simulink model "SBFSRM_CustomModelOK_WindTurbine_1Hp"  (Simulink 8.1)
settings: Solver=ode45  StartTime=0.0  StopTime=0.5  FixedStep=Ts  MaxStep=1e-6  MinStep=1e-7  RelTol=1e-5
values from neighbouring files (symbols this model uses):
  Bm = 0.02    [WorkSpaceBackup1.mat]
  J = 0.048    [WorkSpaceBackup1.mat]
  R = 0.05    [WorkSpaceBackup1.mat]
  Ts = 1e-06    [WorkSpaceBackup1.mat]
undefined symbols (not defined in the file or in its folder): DiscIntNeverNeededParam, find_system, InductanceTest, TorqueTest
libraries: powerlib x49, powerlib_extras x2, simulink x2, dspsigops x1
settings Model: Creator=Rahul  LastModifiedBy=USER
settings DataIOCC: SignalLoggingName=signout
settings OptimizationCC: InitFltsAndDblsToZero=on
settings DebuggingCC: CheckExecutionContextPreStartOutputMsg=on  CheckExecutionContextRuntimeOutputMsg=on  SolverPrmCheckMsg=none  MultiTaskDSMMsg=warning  MultiTaskCondExecSysMsg=none
settings HardwareCC: TargetHWDeviceType=32-bit Generic

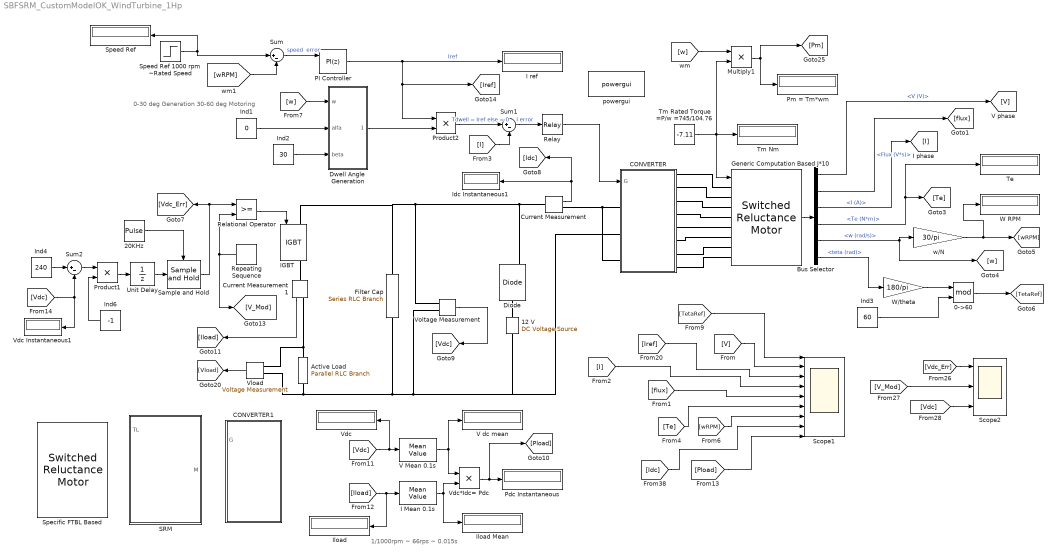
== system SBFSRM_CustomModelOK_WindTurbine_1Hp ==
  note: 1/1000rpm ~ 66rps ~ 0.015s
  note: 0-30 deg Generation
      | 30-60 deg Motoring
  0->60 : Math  Operator=mod  SampleTime=Ts  SaturateOnIntegerOverflow=on
  12 V : powerlib/Electrical Sources/DC Voltage Source  Amplitude=200  Measurements=None
  20KHz : DiscretePulseGenerator  PulseType=Time based  Period=0.5e-4  PulseWidth=10
  Active Load : powerlib/Elements/Parallel RLC Branch  LConnTagsString=a  RConnTagsString=__new0  BranchType=R  Resistance=1  Inductance=1e-3  SetiL0=off  InitialCurrent=0  Capacitance=1e-6  Setx0=off  InitialVoltage=0  Measurements=None
  Bus Selector : BusSelector  OutputSignals=V (V),Flux (V*s),I (A),Te (N*m),w (rad/s),teta (rad)
  CONVERTER : Subsystem  LoadFcn=find_system(gcs,'FollowLinks', 'on', 'LookUnderMasks', 'all');
  CONVERTER1 : Subsystem  LoadFcn=find_system(gcs,'FollowLinks', 'on', 'LookUnderMasks', 'all');
  Current Measurement : powerlib/Measurements/Current Measurement  PhasorSimulation=off  OutputType=Complex  PSBequivalent=0
  Current Measurement1 : powerlib/Measurements/Current Measurement  PhasorSimulation=off  OutputType=Complex  PSBequivalent=0
  Diode : powerlib/Power Electronics/Diode  Ron=0.001  Lon=0  Vf=0.8  IC=0  UseSnubber=off  Rs=10e6  Cs=inf  Measurements=on
  Dwell Angle  Generation : Subsystem
  Filter Cap : powerlib/Elements/Series RLC Branch  LConnTagsString=__new0  RConnTagsString=__new0  BranchType=RC  Resistance=0.001  Inductance=1e-3  SetiL0=off  InitialCurrent=0  Capacitance=3000e-6  Setx0=off  InitialVoltage=0  Measurements=None
  "Generic Computation Based J*10 " : powerlib/Machines/Switched Reluctance Motor  MachineType=8/6  MachineModel=Generic model  StatorResistance=0.013  PlotCurves=off  Inertia=0.0004  Friction=0  InitialSpeed=[97 0]  Lq=0.005  Ld=0.053  Lsat=0.002  MaximumCurrent=20  MaximumFluxLinkage=0.3  MagnetisationCharacteristic='srm64_60kw.mat'  RotorAngleVector=[0 10 20 30 40 45]  StatorCurrentVector=0:25:450  TsPowergui=0  TsBlock=-1
  I Mean 0.1s : powerlib_extras/Measurements/Mean Value  Period=0.015
  I ref : Display
  IGBT : powerlib/Power Electronics/IGBT  Ron=0.001  Lon=0  Vf=1  Tf=1e-6  Tt=2e-6  IC=0  Rs=1e5  Cs=inf  Measurements=on
  Idc Instantaneous1 : Display
  "Iload " : Display
  Iload Mean : Display
  Ind1 : Constant  Value=0
  Ind2 : Constant  Value=30
  Ind3 : Constant  Value=60
  Ind4 : Constant  Value=240
  Ind6 : Constant  Value=-1
  Multiply1 : Product  Inputs=**
  PI Controller : simulink/Continuous/PID Controller  Controller=PI  TimeDomain=Discrete-time  SampleTime=Ts  IntegratorMethod=Trapezoidal  FilterMethod=Forward Euler  Form=Parallel  P=-2  I=-0.1  D=0  N=100  InitialConditionSource=external  InitialConditionForIntegrator=0  InitialConditionForFilter=0  ExternalReset=none  LimitOutput=on  UpperSaturationLimit=20  LowerSaturationLimit=0  LinearizeAsGain=off  AntiWindupMode=clamping  Kb=1  TrackingMode=off  Kt=1  PParamMin=[]  PParamMax=[]  IParamMin=[]  IParamMax=[]  DParamMin=[]  DParamMax=[]  NParamMin=[]  NParamMax=[]  KbParamMin=[]  KbParamMax=[]  KtParamMin=[]  KtParamMax=[]  POutMin=[]  POutMax=[]  IOutMin=[]  IOutMax=[]  DOutMin=[]  DOutMax=[]  NOutMin=[]  NOutMax=[]  KbOutMin=[]  KbOutMax=[]  KtOutMin=[]  KtOutMax=[]  IntegratorOutMin=[]  IntegratorOutMax=[]  FilterOutMin=[]  FilterOutMax=[]  SumOutMin=[]  SumOutMax=[]  SumI1OutMin=[]  SumI1OutMax=[]  SumI2OutMin=[]  SumI2OutMax=[]  SumI3OutMin=[]  SumI3OutMax=[]  SumDOutMin=[]  SumDOutMax=[]  SaturationOutMin=[]  SaturationOutMax=[]  IntegratorContinuousStateAttributes=''  IntegratorStateMustResolveToSignalObject=off  IntegratorRTWStateStorageClass=Auto  FilterContinuousStateAttributes=''  FilterStateMustResolveToSignalObject=off  FilterRTWStateStorageClass=Auto
  Pdc Instantaneous : Display
  Pm = Tm*wm : Display
  Product1 : Product
  Product2 : Product  RndMeth=Zero
  Relational Operator : RelationalOperator  OutDataTypeStr=boolean
  Relay : Relay  OnSwitchValue=0.1  OffSwitchValue=-0.1
  Repeating Sequence : simulink/Sources/Repeating Sequence  rep_seq_t=[0 0.25e-4 0.5e-4]  rep_seq_y=[0 1 0]
  SRM : Subsystem
  Sample and Hold : dspsigops/Sample and Hold  trig=Rising edge  initCond=0  latchinput=off
  Scope1 : Scope  NumInputPorts=9
      settings: TimeRange=0.1400000000000001  YMin=0~-300~0~-5~-0.1~-10~0~-250~0  YMax=100~300~12~20~0.4~10~1200~250~800  SaveName=ScopeData2  MaxDataPoints=100000
  Scope2 : Scope  NumInputPorts=3
      settings: TimeRange=0.1400000000000001  YMin=-5~-2~0  YMax=5~2~300  MaxDataPoints=100000
  Specific FTBL Based : powerlib/Machines/Switched Reluctance Motor  MachineType=6/4  MachineModel=Specific model  StatorResistance=R  PlotCurves=off  Inertia=J  Friction=Bm  InitialSpeed=[355 0]  Lq=0.67e-3  Ld=23.6e-3  Lsat=0.15e-3  MaximumCurrent=450  MaximumFluxLinkage=0.486  MagnetisationCharacteristic='SRM64StandardTables.mat'  RotorAngleVector=[0,1,2,3,4,5,6,7,8,9,10,11,12,13,14,15,16,17,18,19,20,21,22,23,24,25,26,27,28,29,30,31,32,33,34,35,36,37,38,39,40,41,42,43,44,45,46,47,48,49,50,51,52,53,54,55,56,57,58,59,60,61,62,63,64,65,66,67,68,69,70,71,72,73,74,75,76,77,78,79,80,81,82,83,84,85,86,87,88,89,90]  StatorCurrentVector=[0,0.1,0.3,0.5,0.7,0.9,1,2,3,4,5,6,7,8,9,10,11,12,13,14,15,16,17,18,19,20,21,22,23,24,25,26,27,28,29,30,31,32,33,34,35,36,37,38,39,40,41,42,43,44,45,46,47,48,49,50,51,52,53,54,55,56,57,58,59,60,61,62,63,64,65,66,67,68,69,70,71,72,73,74,75,76,77,78,79,80,81,82,83,84,85,86,87,88,89,90,91,92,93,94,95,96,97,98,99,100,101,102,103,104,105,106,107,108,109,110,111,112,113,114,115,116,117,118,119,120,121,122,123,124,125,126,127,128,129,130,131,132,133,134,135,136,137,138,139,140,141,142,143,144,145,146,147,148,149,150,151,152,153,154,155,156,157,158,159,160,161,162,163,164,165,166,167,168]  TsPowergui=0  TsBlock=-1
  Speed Ref : Display
  Speed Ref 1000 rpm ~Rated Speed : Step  Time=0.1  Before=1000  After=1000  SampleTime=0
  Sum : Sum  Inputs=|+-
  Sum1 : Sum  Inputs=|+-
  Sum2 : Sum  Inputs=|+-
  Te : Display
  Tm Nm : Display
  Tm Rated Torque =P/w =745/104.76 : Constant  Value=-7.11
  Unit Delay : UnitDelay  SampleTime=-1
  V Mean 0.1s : powerlib_extras/Measurements/Mean Value  Period=0.015
  V dc mean : Display
  "Vdc " : Display
  Vdc Instantaneous1 : Display
  Vdc*Idc= Pdc : Product
  Vload : powerlib/Measurements/Voltage Measurement  PhasorSimulation=off  OutputType=Complex  PSBequivalent=0
  Voltage Measurement : powerlib/Measurements/Voltage Measurement  PhasorSimulation=off  OutputType=Complex  PSBequivalent=0
  W RPM : Display
  W/theta : Gain  Gain=180/pi
  powergui : powerlib/powergui  Priority=1  SimulationMode=Discrete  SolverType=Tustin  SampleTime=Ts  frequency=60  SPID=off  DisableSnubberDevices=off  DisableRonSwitches=off  DisableVfSwitches=off  SwTol=0  Interpol=off  DisplayEquations=off  frequencyindice=0  Pbase=100e6  ErrMax=1e-4  Iterations=50  UnitsV=kV  UnitsW=MW  FunctionMessages=off  echomessages=off  HookPort=off  EnableUseOfTLC=off  x0status=blocks  RestoreLinks=warning  ResistiveCurrentMeasurement=off  Frange=[0:2:500]  Ylog=off  Xlog=on  ShowGrid=off  save=off  variable=ZData  ZoomFFT=off  StartTime=0.0  cycles=1  DisplayStyle=1  fundamental=60  FreqAxis=off  MaxFrequency=1000  frequencyindicesteady=1  RmsSteady=1  display=off  Ts=0  methode=off
  w/N : Gain  Gain=30/pi
  wires:
  Sum1/1 -> Relay/1  "I error"
  Relay/1 -> CONVERTER/1(G)
  Product2/1 -> Sum1/1  "Tdwell = Iref else = 0"
  "Generic Computation Based J*10 "/1 -> Bus Selector/1
  Bus Selector/6 -> W/theta/1  "<teta (rad)>"
  w/N/1 -> [wRPM], W RPM/1
  Ind3/1 -> 0->60/2
  W/theta/1 -> 0->60/1
  Bus Selector/1 -> [V]  "<V (V)>"
  Bus Selector/2 -> [flux]  "<Flux (V*s)>"
  Bus Selector/3 -> [I]  "<I (A)>"
  [I] -> Sum1/2
  Bus Selector/4 -> [Te], Te/1  "<Te (N*m)>"
  Bus Selector/5 -> w/N/1, [w]  "<w (rad/s)>"
  0->60/1 -> [TetaRef]
  Voltage Measurement/1 -> [Vdc]
  Current Measurement/1 -> Idc Instantaneous1/1, [Idc]
  [Iload] -> I Mean 0.1s/1, "Iload "/1
  Ind4/1 -> Sum2/1
  [Vdc] -> Sum2/2, Vdc Instantaneous1/1
  Vdc*Idc= Pdc/1 -> [Pload], Pdc Instantaneous/1
  Current Measurement1/1 -> [Iload]
  [w] -> Multiply1/1
  Multiply1/1 -> [Pm], Pm = Tm*wm/1
  Tm Rated Torque =P/w =745/104.76/1 -> Tm Nm/1, "Generic Computation Based J*10 "/1, Multiply1/2
  Repeating Sequence/1 -> Relational Operator/2, [V_Mod]
  Relational Operator/1 -> IGBT/1
  Sum2/1 -> Product1/1
  Ind6/1 -> Product1/2
  Product1/1 -> Unit Delay/1
  Unit Delay/1 -> Sample and Hold/1
  Sample and Hold/1 -> Relational Operator/1, [Vdc_Err]
  20KHz/1 -> Sample and Hold/Trigger
  [Vdc] -> V Mean 0.1s/1, "Vdc "/1
  I Mean 0.1s/1 -> Iload Mean/1, Vdc*Idc= Pdc/2
  Vload/1 -> [Vload]
  V Mean 0.1s/1 -> V dc mean/1, Vdc*Idc= Pdc/1
  Ind1/1 -> Dwell Angle  Generation/2(alfa)
  Ind2/1 -> Dwell Angle  Generation/3(beta)
  [w] -> Dwell Angle  Generation/1(w)
  Dwell Angle  Generation/1(Signal) -> Product2/2
  [TetaRef] -> Scope1/1
  [V] -> Scope1/2
  [Iref] -> Scope1/3
  [I] -> Scope1/4
  [Pload] -> Scope1/9
  [Idc] -> Scope1/8
  [wRPM] -> Scope1/7
  [Te] -> Scope1/6
  [flux] -> Scope1/5
  [Vdc_Err] -> Scope2/1
  [V_Mod] -> Scope2/2
  [Vdc] -> Scope2/3
  Sum/1 -> PI Controller/1  "speed  error"
  Speed Ref 1000 rpm ~Rated Speed/1 -> Sum/1, Speed Ref/1
  [wRPM] -> Sum/2
  PI Controller/1 -> Product2/1, [Iref], I ref/1  "Iref"
  connections:
  "Generic Computation Based J*10 "/LConn1 -- CONVERTER/RConn1
  "Generic Computation Based J*10 "/LConn2 -- CONVERTER/RConn2
  "Generic Computation Based J*10 "/LConn3 -- CONVERTER/RConn3
  "Generic Computation Based J*10 "/LConn4 -- CONVERTER/RConn4
  "Generic Computation Based J*10 "/LConn5 -- CONVERTER/RConn5
  "Generic Computation Based J*10 "/LConn6 -- CONVERTER/RConn6
  Voltage Measurement/LConn2 -- Vload/LConn2 -- Active Load/RConn1 -- Filter Cap/RConn1 -- CONVERTER/LConn2 -- 12 V/LConn1
  Current Measurement/LConn1 -- Filter Cap/LConn1 -- IGBT/LConn1 -- Voltage Measurement/LConn1 -- Diode/RConn1
  Current Measurement/RConn1 -- CONVERTER/LConn3 -- CONVERTER/LConn1
  Diode/LConn1 -- 12 V/RConn1
  Active Load/LConn1 -- Vload/LConn1 -- Current Measurement1/RConn1
  IGBT/RConn1 -- Current Measurement1/LConn1
  CONVERTER/RConn7 -- "Generic Computation Based J*10 "/LConn7
  CONVERTER/RConn8 -- "Generic Computation Based J*10 "/LConn8

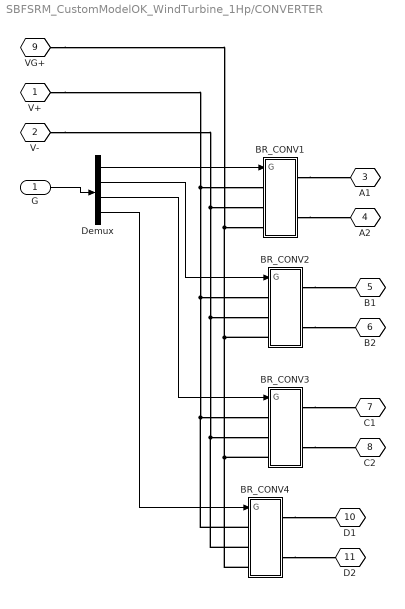
== system SBFSRM_CustomModelOK_WindTurbine_1Hp/CONVERTER ==
  G : Inport
  BR_CONV1 : Subsystem
  BR_CONV2 : Subsystem
  BR_CONV3 : Subsystem
  BR_CONV4 : Subsystem
  Demux : Demux
  V+ : PMIOPort  Tag=PMCPort  Port=1  Side=Left
  V- : PMIOPort  Tag=PMCPort  Port=2  Side=Left
  A1 : PMIOPort  Tag=PMCPort  Port=3  Side=Right
  A2 : PMIOPort  Tag=PMCPort  Port=4  Side=Right
  B1 : PMIOPort  Tag=PMCPort  Port=5  Side=Right
  B2 : PMIOPort  Tag=PMCPort  Port=6  Side=Right
  C1 : PMIOPort  Tag=PMCPort  Port=7  Side=Right
  C2 : PMIOPort  Tag=PMCPort  Port=8  Side=Right
  VG+ : PMIOPort  Tag=PMCPort  Port=9  Side=Left
  D1 : PMIOPort  Tag=PMCPort  Port=10  Side=Right
  D2 : PMIOPort  Tag=PMCPort  Port=11  Side=Right
  wires:
  Demux/3 -> BR_CONV3/1(G)
  Demux/1 -> BR_CONV1/1(G)
  G/1 -> Demux/1
  Demux/2 -> BR_CONV2/1(G)
  Demux/4 -> BR_CONV4/1(G)
  connections:
  BR_CONV3/RConn2 -- C2/RConn1
  BR_CONV3/RConn1 -- C1/RConn1
  BR_CONV2/RConn2 -- B2/RConn1
  BR_CONV2/RConn1 -- B1/RConn1
  BR_CONV1/RConn2 -- A2/RConn1
  BR_CONV1/RConn1 -- A1/RConn1
  BR_CONV1/LConn2 -- V-/RConn1 -- BR_CONV4/LConn2 -- BR_CONV3/LConn2 -- BR_CONV2/LConn2
  V+/RConn1 -- BR_CONV1/LConn1 -- BR_CONV4/LConn1 -- BR_CONV3/LConn1 -- BR_CONV2/LConn1
  VG+/RConn1 -- BR_CONV1/LConn3 -- BR_CONV4/LConn3 -- BR_CONV3/LConn3 -- BR_CONV2/LConn3
  BR_CONV4/RConn2 -- D2/RConn1
  BR_CONV4/RConn1 -- D1/RConn1

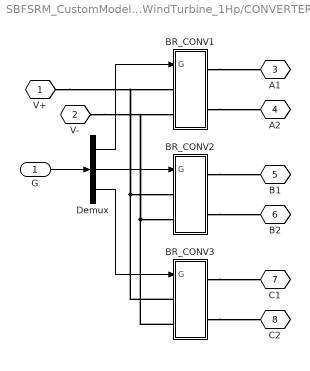
== system SBFSRM_CustomModelOK_WindTurbine_1Hp/CONVERTER1 ==
  G : Inport
  BR_CONV1 : Subsystem
  BR_CONV2 : Subsystem
  BR_CONV3 : Subsystem
  Demux : Demux  Outputs=3
  V+ : PMIOPort  Tag=PMCPort  Port=1  Side=Left
  V- : PMIOPort  Tag=PMCPort  Port=2  Side=Left
  A1 : PMIOPort  Tag=PMCPort  Port=3  Side=Right
  A2 : PMIOPort  Tag=PMCPort  Port=4  Side=Right
  B1 : PMIOPort  Tag=PMCPort  Port=5  Side=Right
  B2 : PMIOPort  Tag=PMCPort  Port=6  Side=Right
  C1 : PMIOPort  Tag=PMCPort  Port=7  Side=Right
  C2 : PMIOPort  Tag=PMCPort  Port=8  Side=Right
  wires:
  Demux/3 -> BR_CONV3/1(G)
  Demux/1 -> BR_CONV1/1(G)
  Demux/2 -> BR_CONV2/1(G)
  G/1 -> Demux/1
  connections:
  BR_CONV3/RConn2 -- C2/RConn1
  BR_CONV3/RConn1 -- C1/RConn1
  BR_CONV2/RConn2 -- B2/RConn1
  BR_CONV2/RConn1 -- B1/RConn1
  BR_CONV1/RConn2 -- A2/RConn1
  BR_CONV1/RConn1 -- A1/RConn1
  BR_CONV3/LConn2 -- BR_CONV1/LConn2 -- V-/RConn1 -- BR_CONV2/LConn2
  BR_CONV3/LConn1 -- BR_CONV1/LConn1 -- V+/RConn1 -- BR_CONV2/LConn1

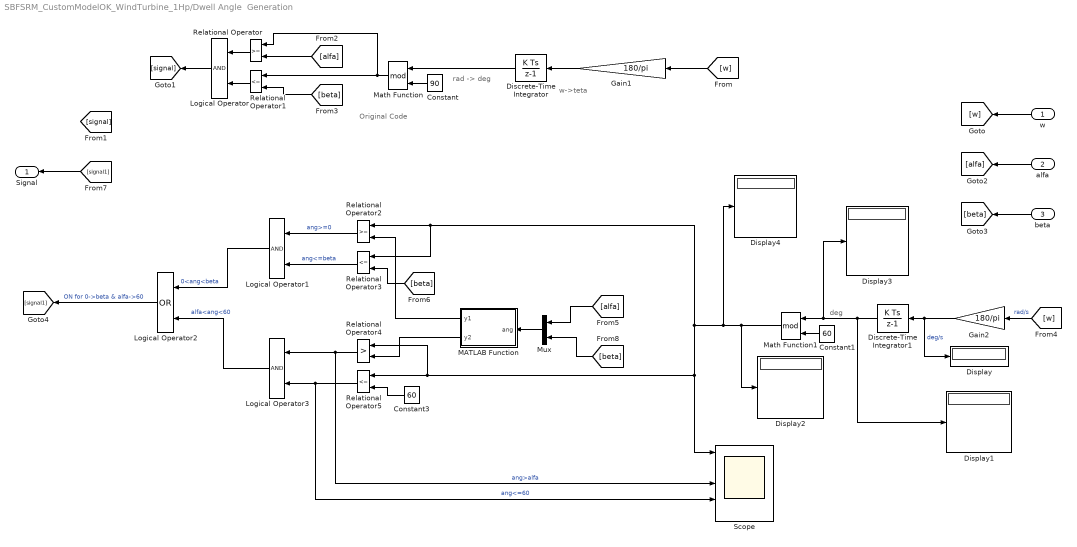
== system SBFSRM_CustomModelOK_WindTurbine_1Hp/Dwell Angle  Generation ==
  note: Original Code
  note: rad -> deg
  note: w->teta
  note: deg
  w : Inport
  alfa : Inport  Port=2
  beta : Inport  Port=3
  Constant : Constant  Value=90
  Constant1 : Constant  Value=60
  Constant3 : Constant  Value=60
  Discrete-Time Integrator : DiscreteIntegrator  InitialCondition=[0 -30 -60]  SampleTime=Ts  ICPrevOutput=DiscIntNeverNeededParam  ICPrevScaledInput=DiscIntNeverNeededParam
  Discrete-Time Integrator1 : DiscreteIntegrator  InitialCondition=[0 -15 -30 -45]  SampleTime=Ts  ICPrevOutput=DiscIntNeverNeededParam  ICPrevScaledInput=DiscIntNeverNeededParam
  Display{,1..4} (5 alike) : Display
  Gain1 : Gain  Gain=180/pi  SaturateOnIntegerOverflow=on  OutDataTypeStr=Inherit: Same as input  ParamDataTypeStr=Inherit: Same as input
  Gain2 : Gain  Gain=180/pi  SaturateOnIntegerOverflow=on  OutDataTypeStr=Inherit: Same as input  ParamDataTypeStr=Inherit: Same as input
  Logical Operator : Logic  AllPortsSameDT=off
  Logical Operator1 : Logic  AllPortsSameDT=off
  Logical Operator2 : Logic  Operator=OR  AllPortsSameDT=off
  Logical Operator3 : Logic  AllPortsSameDT=off
  MATLAB Function : MATLAB Function  TreatAsAtomicUnit=on
  Math Function : Math  Operator=mod  SaturateOnIntegerOverflow=on
  Math Function1 : Math  Operator=mod  SaturateOnIntegerOverflow=on
  Mux : Mux  Inputs=2
  Relational Operator : RelationalOperator
  Relational Operator1 : RelationalOperator  Operator=<=
  Relational Operator2 : RelationalOperator
  Relational Operator3 : RelationalOperator  Operator=<=
  Relational Operator4 : RelationalOperator  Operator=>
  Relational Operator5 : RelationalOperator  Operator=<=
  Scope : Scope  NumInputPorts=5
      settings: YMin=-5~-5~-5~-5~-5  YMax=5~5~5~5~5
  Signal : Outport
  wires:
  Math Function/1 -> Relational Operator/1, Relational Operator1/1
  Relational Operator1/1 -> Logical Operator/2
  beta/1 -> [beta]
  alfa/1 -> [alfa]
  Relational Operator/1 -> Logical Operator/1
  Constant/1 -> Math Function/2
  Logical Operator/1 -> [signal]
  Discrete-Time Integrator/1 -> Math Function/1
  Gain1/1 -> Discrete-Time Integrator/1
  w/1 -> [w]
  [w] -> Gain2/1  "rad/s"
  Math Function1/1 -> Display2/1, Relational Operator3/1, Relational Operator2/1, Scope/1, Relational Operator4/1, Relational Operator5/1, Display4/1
  Gain2/1 -> Display/1, Discrete-Time Integrator1/1  "deg/s"
  [beta] -> Relational Operator3/2
  Relational Operator2/1 -> Logical Operator1/1  "ang>=0"
  Constant1/1 -> Math Function1/2
  Discrete-Time Integrator1/1 -> Display1/1, Math Function1/1, Display3/1
  Relational Operator3/1 -> Logical Operator1/2  "ang<=beta"
  Logical Operator1/1 -> Logical Operator2/1  "0<ang<beta"
  Logical Operator3/1 -> Logical Operator2/2  "alfa<ang<60"
  Logical Operator2/1 -> [signal1]  "ON for 0->beta & alfa->60"
  Constant3/1 -> Relational Operator5/2
  Relational Operator4/1 -> Scope/3, Logical Operator3/1  "ang>alfa"
  Relational Operator5/1 -> Scope/4, Logical Operator3/2  "ang<=60"
  MATLAB Function/1(y1) -> Relational Operator2/2
  Mux/1 -> MATLAB Function/1(ang)
  [alfa] -> Mux/1
  [w] -> Gain1/1
  [alfa] -> Relational Operator/2
  [beta] -> Relational Operator1/2
  [signal1] -> Signal/1
  [beta] -> Mux/2
  MATLAB Function/2(y2) -> Relational Operator4/2

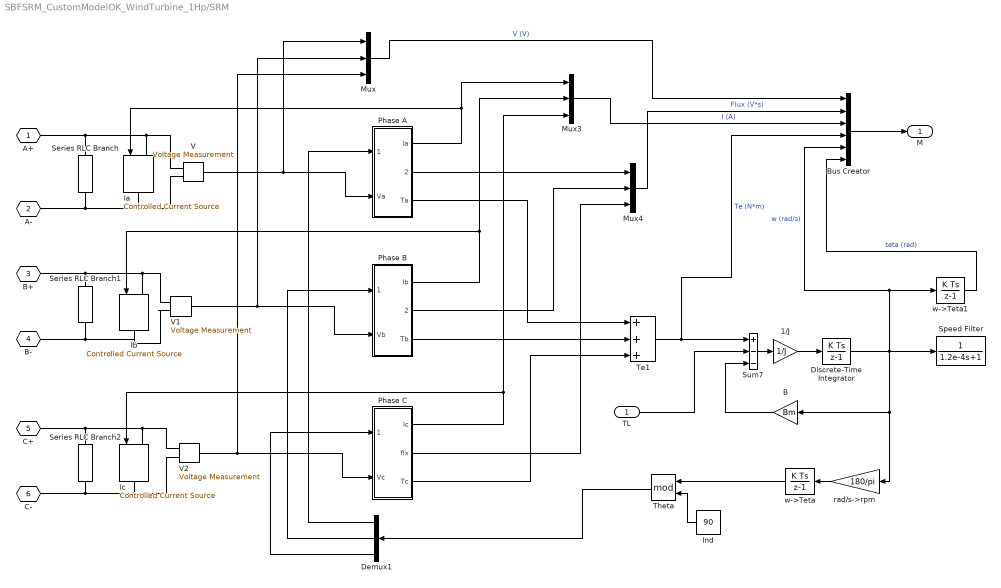
== system SBFSRM_CustomModelOK_WindTurbine_1Hp/SRM ==
  TL : Inport
  1/J : Gain  Gain=1/J  SaturateOnIntegerOverflow=on  OutDataTypeStr=Inherit: Same as input  ParamDataTypeStr=Inherit: Same as input
  B : Gain  Gain=Bm  SaturateOnIntegerOverflow=on  OutDataTypeStr=Inherit: Same as input  ParamDataTypeStr=Inherit: Same as input
  Bus Creator : BusCreator  Inputs=6
  Demux1 : Demux  Outputs=3
  Discrete-Time Integrator : DiscreteIntegrator  InitialCondition=305  SampleTime=Ts  ICPrevOutput=DiscIntNeverNeededParam  ICPrevScaledInput=DiscIntNeverNeededParam
  Ia : powerlib/Electrical Sources/Controlled Current Source  Initialize=on  Source_Type=DC  Amplitude=0  Phase=0  Frequency=0  Measurements=None
  Ib : powerlib/Electrical Sources/Controlled Current Source  Initialize=on  Source_Type=DC  Amplitude=0  Phase=0  Frequency=0  Measurements=None
  Ic : powerlib/Electrical Sources/Controlled Current Source  Initialize=on  Source_Type=DC  Amplitude=0  Phase=0  Frequency=0  Measurements=None
  Ind : Constant  Value=90
  Mux : Mux  Inputs=3
  Mux3 : Mux  Inputs=3
  Mux4 : Mux  Inputs=3
  Phase A : Subsystem
  Phase B : Subsystem
  Phase C : Subsystem
  Series RLC Branch : powerlib/Elements/Series RLC Branch  LConnTagsString=__new0  RConnTagsString=__new0  BranchType=R  Resistance=10e6  Inductance=1e-3  SetiL0=off  InitialCurrent=0  Capacitance=1e-6  Setx0=off  InitialVoltage=0  Measurements=None
  Series RLC Branch1 : powerlib/Elements/Series RLC Branch  LConnTagsString=__new0  RConnTagsString=__new0  BranchType=R  Resistance=10e6  Inductance=1e-3  SetiL0=off  InitialCurrent=0  Capacitance=1e-6  Setx0=off  InitialVoltage=0  Measurements=None
  Series RLC Branch2 : powerlib/Elements/Series RLC Branch  LConnTagsString=__new0  RConnTagsString=__new0  BranchType=R  Resistance=10e6  Inductance=1e-3  SetiL0=off  InitialCurrent=0  Capacitance=1e-6  Setx0=off  InitialVoltage=0  Measurements=None
  Speed Filter : TransferFcn  Denominator=[1.2e-4 1]
  Sum7 : Sum  Inputs=+--  SaturateOnIntegerOverflow=on
  Te1 : Sum  Inputs=+++
  Theta : Math  Operator=mod  SampleTime=Ts  SaturateOnIntegerOverflow=on
  V : powerlib/Measurements/Voltage Measurement  PhasorSimulation=off  OutputType=Complex  PSBequivalent=0
  V1 : powerlib/Measurements/Voltage Measurement  PhasorSimulation=off  OutputType=Complex  PSBequivalent=0
  V2 : powerlib/Measurements/Voltage Measurement  PhasorSimulation=off  OutputType=Complex  PSBequivalent=0
  rad/s->rpm : Gain  Gain=180/pi
  w->Teta : DiscreteIntegrator  InitialCondition=[0 -30 -60]  SampleTime=Ts  ICPrevOutput=DiscIntNeverNeededParam  ICPrevScaledInput=DiscIntNeverNeededParam
  w->Teta1 : DiscreteIntegrator  InitialCondition=[0 -pi/6 -pi/3]  SampleTime=Ts  ICPrevOutput=DiscIntNeverNeededParam  ICPrevScaledInput=DiscIntNeverNeededParam
  A+ : PMIOPort  Tag=PMCPort  Port=1  Side=Left
  A- : PMIOPort  Tag=PMCPort  Port=2  Side=Left
  B+ : PMIOPort  Tag=PMCPort  Port=3  Side=Left
  B- : PMIOPort  Tag=PMCPort  Port=4  Side=Left
  C+ : PMIOPort  Tag=PMCPort  Port=5  Side=Left
  C- : PMIOPort  Tag=PMCPort  Port=6  Side=Left
  M : Outport
  wires:
  Mux4/1 -> Bus Creator/2  "Flux (V*s)"
  Mux/1 -> Bus Creator/1  "V (V)"
  Phase A/3(Ta) -> Te1/1
  Phase C/3(Tc) -> Te1/3
  Phase B/3(Tb) -> Te1/2
  Phase A/2(flxa) -> Mux4/1
  Phase B/2(flxb) -> Mux4/2
  Phase C/2(flx) -> Mux4/3
  Phase B/1(Ib) -> Ib/1, Mux3/2
  Phase C/1(Ic) -> Mux3/3, Ic/1
  Demux1/1 -> Phase A/1(theta)
  Demux1/3 -> Phase C/1(theta)
  V/1 -> Phase A/2(Va), Mux/1
  V2/1 -> Phase C/2(Vc), Mux/3
  Sum7/1 -> 1/J/1
  B/1 -> Sum7/3
  1/J/1 -> Discrete-Time Integrator/1
  TL/1 -> Sum7/2
  Te1/1 -> Bus Creator/4, Sum7/1  "Te (N*m)"
  Discrete-Time Integrator/1 -> rad/s->rpm/1, B/1, w->Teta1/1, Bus Creator/5, Speed Filter/1  "w (rad/s)"
  Ind/1 -> Theta/2
  Theta/1 -> Demux1/1
  Phase A/1(Ia) -> Ia/1, Mux3/1
  Demux1/2 -> Phase B/1(theta)
  V1/1 -> Phase B/2(Vb), Mux/2
  Mux3/1 -> Bus Creator/3  "I (A)"
  Bus Creator/1 -> M/1
  w->Teta/1 -> Theta/1
  rad/s->rpm/1 -> w->Teta/1
  w->Teta1/1 -> Bus Creator/6  "teta (rad)"
  connections:
  V2/LConn1 -- Series RLC Branch2/LConn1 -- C+/RConn1 -- Ic/LConn1
  Ic/RConn1 -- Series RLC Branch2/RConn1 -- C-/RConn1 -- V2/LConn2
  V1/LConn2 -- Series RLC Branch1/RConn1 -- B-/RConn1 -- Ib/RConn1
  Ib/LConn1 -- Series RLC Branch1/LConn1 -- B+/RConn1 -- V1/LConn1
  V/LConn2 -- Series RLC Branch/RConn1 -- A-/RConn1 -- Ia/RConn1
  V/LConn1 -- Series RLC Branch/LConn1 -- A+/RConn1 -- Ia/LConn1

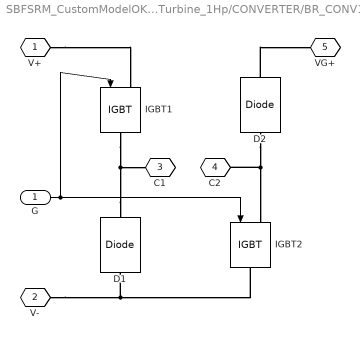
== system SBFSRM_CustomModelOK_WindTurbine_1Hp/CONVERTER/BR_CONV1 ==
  G : Inport
  D1 : powerlib/Power Electronics/Diode  Ron=1e-3  Lon=0  Vf=0.8  IC=0  UseSnubber=off  Rs=10000  Cs=inf  Measurements=off
  D2 : powerlib/Power Electronics/Diode  Ron=1e-3  Lon=0  Vf=0.8  IC=0  UseSnubber=off  Rs=10000  Cs=inf  Measurements=off
  IGBT1 : powerlib/Power Electronics/IGBT  Ron=1e-3  Lon=0  Vf=1  Tf=0  Tt=0  IC=0  Rs=2000  Cs=0.1e-6  Measurements=off
  IGBT2 : powerlib/Power Electronics/IGBT  Ron=1e-3  Lon=0  Vf=1  Tf=0  Tt=0  IC=0  Rs=2000  Cs=0.1e-6  Measurements=off
  V+ : PMIOPort  Tag=PMCPort  Port=1  Side=Left
  V- : PMIOPort  Tag=PMCPort  Port=2  Side=Left
  C1 : PMIOPort  Tag=PMCPort  Port=3  Side=Right
  C2 : PMIOPort  Tag=PMCPort  Port=4  Side=Right
  VG+ : PMIOPort  Tag=PMCPort  Port=5  Side=Left
  wires:
  G/1 -> IGBT1/1, IGBT2/1
  connections:
  D1/LConn1 -- V-/RConn1 -- IGBT2/RConn1
  D2/LConn1 -- IGBT2/LConn1 -- C2/RConn1
  D1/RConn1 -- IGBT1/RConn1 -- C1/RConn1
  V+/RConn1 -- IGBT1/LConn1
  D2/RConn1 -- VG+/RConn1

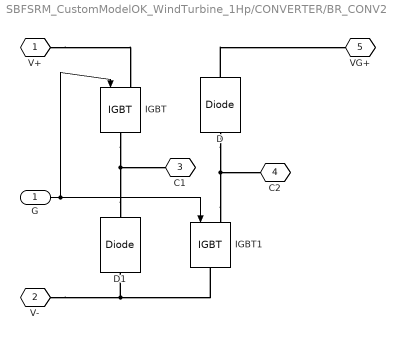
== system SBFSRM_CustomModelOK_WindTurbine_1Hp/CONVERTER/BR_CONV2 ==
  G : Inport
  D : powerlib/Power Electronics/Diode  Ron=1e-3  Lon=0  Vf=0.8  IC=0  UseSnubber=off  Rs=10000  Cs=inf  Measurements=off
  D1 : powerlib/Power Electronics/Diode  Ron=1e-3  Lon=0  Vf=0.8  IC=0  UseSnubber=off  Rs=10000  Cs=inf  Measurements=off
  IGBT : powerlib/Power Electronics/IGBT  Ron=1e-3  Lon=0  Vf=1  Tf=0  Tt=0  IC=0  Rs=2000  Cs=0.1e-6  Measurements=off
  IGBT1 : powerlib/Power Electronics/IGBT  Ron=1e-3  Lon=0  Vf=1  Tf=0  Tt=0  IC=0  Rs=2000  Cs=0.1e-6  Measurements=off
  V+ : PMIOPort  Tag=PMCPort  Port=1  Side=Left
  V- : PMIOPort  Tag=PMCPort  Port=2  Side=Left
  C1 : PMIOPort  Tag=PMCPort  Port=3  Side=Right
  C2 : PMIOPort  Tag=PMCPort  Port=4  Side=Right
  VG+ : PMIOPort  Tag=PMCPort  Port=5  Side=Left
  wires:
  G/1 -> IGBT/1, IGBT1/1
  connections:
  D1/LConn1 -- V-/RConn1 -- IGBT1/RConn1
  IGBT1/LConn1 -- D/LConn1 -- C2/RConn1
  D1/RConn1 -- IGBT/RConn1 -- C1/RConn1
  V+/RConn1 -- IGBT/LConn1
  D/RConn1 -- VG+/RConn1

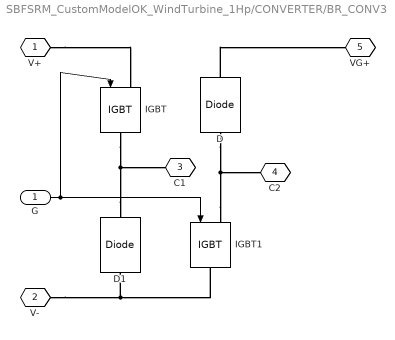
== system SBFSRM_CustomModelOK_WindTurbine_1Hp/CONVERTER/BR_CONV3 ==
  G : Inport
  D : powerlib/Power Electronics/Diode  Ron=1e-3  Lon=0  Vf=0.8  IC=0  UseSnubber=off  Rs=10000  Cs=inf  Measurements=off
  D1 : powerlib/Power Electronics/Diode  Ron=1e-3  Lon=0  Vf=0.8  IC=0  UseSnubber=off  Rs=10000  Cs=inf  Measurements=off
  IGBT : powerlib/Power Electronics/IGBT  Ron=1e-3  Lon=0  Vf=1  Tf=0  Tt=0  IC=0  Rs=2000  Cs=0.1e-6  Measurements=off
  IGBT1 : powerlib/Power Electronics/IGBT  Ron=1e-3  Lon=0  Vf=1  Tf=0  Tt=0  IC=0  Rs=2000  Cs=0.1e-6  Measurements=off
  V+ : PMIOPort  Tag=PMCPort  Port=1  Side=Left
  V- : PMIOPort  Tag=PMCPort  Port=2  Side=Left
  C1 : PMIOPort  Tag=PMCPort  Port=3  Side=Right
  C2 : PMIOPort  Tag=PMCPort  Port=4  Side=Right
  VG+ : PMIOPort  Tag=PMCPort  Port=5  Side=Left
  wires:
  G/1 -> IGBT/1, IGBT1/1
  connections:
  D1/LConn1 -- V-/RConn1 -- IGBT1/RConn1
  IGBT1/LConn1 -- D/LConn1 -- C2/RConn1
  D1/RConn1 -- IGBT/RConn1 -- C1/RConn1
  V+/RConn1 -- IGBT/LConn1
  D/RConn1 -- VG+/RConn1

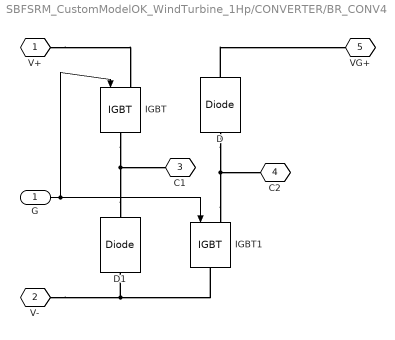
== system SBFSRM_CustomModelOK_WindTurbine_1Hp/CONVERTER/BR_CONV4 ==
  G : Inport
  D : powerlib/Power Electronics/Diode  Ron=1e-3  Lon=0  Vf=0.8  IC=0  UseSnubber=off  Rs=10000  Cs=inf  Measurements=off
  D1 : powerlib/Power Electronics/Diode  Ron=1e-3  Lon=0  Vf=0.8  IC=0  UseSnubber=off  Rs=10000  Cs=inf  Measurements=off
  IGBT : powerlib/Power Electronics/IGBT  Ron=1e-3  Lon=0  Vf=1  Tf=0  Tt=0  IC=0  Rs=2000  Cs=0.1e-6  Measurements=off
  IGBT1 : powerlib/Power Electronics/IGBT  Ron=1e-3  Lon=0  Vf=1  Tf=0  Tt=0  IC=0  Rs=2000  Cs=0.1e-6  Measurements=off
  V+ : PMIOPort  Tag=PMCPort  Port=1  Side=Left
  V- : PMIOPort  Tag=PMCPort  Port=2  Side=Left
  C1 : PMIOPort  Tag=PMCPort  Port=3  Side=Right
  C2 : PMIOPort  Tag=PMCPort  Port=4  Side=Right
  VG+ : PMIOPort  Tag=PMCPort  Port=5  Side=Left
  wires:
  G/1 -> IGBT/1, IGBT1/1
  connections:
  D1/LConn1 -- V-/RConn1 -- IGBT1/RConn1
  IGBT1/LConn1 -- D/LConn1 -- C2/RConn1
  D1/RConn1 -- IGBT/RConn1 -- C1/RConn1
  V+/RConn1 -- IGBT/LConn1
  D/RConn1 -- VG+/RConn1

== system SBFSRM_CustomModelOK_WindTurbine_1Hp/CONVERTER1/BR_CONV1 ==
  G : Inport
  D : powerlib/Power Electronics/Diode  Ron=1e-3  Lon=0  Vf=0.8  IC=0  UseSnubber=off  Rs=1000  Cs=inf  Measurements=off
  D1 : powerlib/Power Electronics/Diode  Ron=1e-3  Lon=0  Vf=0.8  IC=0  UseSnubber=off  Rs=1000  Cs=inf  Measurements=off
  IGBT : powerlib/Power Electronics/IGBT  Ron=1e-3  Lon=0  Vf=1  Tf=0  Tt=0  IC=0  Rs=200  Cs=0.1e-6  Measurements=off
  IGBT1 : powerlib/Power Electronics/IGBT  Ron=1e-3  Lon=0  Vf=1  Tf=0  Tt=0  IC=0  Rs=200  Cs=0.1e-6  Measurements=off
  V+ : PMIOPort  Tag=PMCPort  Port=1  Side=Left
  V- : PMIOPort  Tag=PMCPort  Port=2  Side=Left
  C1 : PMIOPort  Tag=PMCPort  Port=3  Side=Right
  C2 : PMIOPort  Tag=PMCPort  Port=4  Side=Right
  wires:
  G/1 -> IGBT/1, IGBT1/1
  connections:
  D1/LConn1 -- V-/RConn1 -- IGBT1/RConn1
  IGBT1/LConn1 -- D/LConn1 -- C2/RConn1
  D1/RConn1 -- IGBT/RConn1 -- C1/RConn1
  D/RConn1 -- V+/RConn1 -- IGBT/LConn1

== system SBFSRM_CustomModelOK_WindTurbine_1Hp/CONVERTER1/BR_CONV2 ==
  G : Inport
  D : powerlib/Power Electronics/Diode  Ron=1e-3  Lon=0  Vf=0.8  IC=0  UseSnubber=off  Rs=1000  Cs=inf  Measurements=off
  D1 : powerlib/Power Electronics/Diode  Ron=1e-3  Lon=0  Vf=0.8  IC=0  UseSnubber=off  Rs=1000  Cs=inf  Measurements=off
  IGBT : powerlib/Power Electronics/IGBT  Ron=1e-3  Lon=0  Vf=1  Tf=0  Tt=0  IC=0  Rs=200  Cs=0.1e-6  Measurements=off
  IGBT1 : powerlib/Power Electronics/IGBT  Ron=1e-3  Lon=0  Vf=1  Tf=0  Tt=0  IC=0  Rs=200  Cs=0.1e-6  Measurements=off
  V+ : PMIOPort  Tag=PMCPort  Port=1  Side=Left
  V- : PMIOPort  Tag=PMCPort  Port=2  Side=Left
  C1 : PMIOPort  Tag=PMCPort  Port=3  Side=Right
  C2 : PMIOPort  Tag=PMCPort  Port=4  Side=Right
  wires:
  G/1 -> IGBT1/1, IGBT/1
  connections:
  IGBT/LConn1 -- V+/RConn1 -- D/RConn1
  IGBT/RConn1 -- D1/RConn1 -- C1/RConn1
  D/LConn1 -- IGBT1/LConn1 -- C2/RConn1
  V-/RConn1 -- D1/LConn1 -- IGBT1/RConn1

== system SBFSRM_CustomModelOK_WindTurbine_1Hp/CONVERTER1/BR_CONV3 ==
  G : Inport
  D : powerlib/Power Electronics/Diode  Ron=1e-3  Lon=0  Vf=0.8  IC=0  UseSnubber=off  Rs=1000  Cs=inf  Measurements=off
  D1 : powerlib/Power Electronics/Diode  Ron=1e-3  Lon=0  Vf=0.8  IC=0  UseSnubber=off  Rs=1000  Cs=inf  Measurements=off
  IGBT : powerlib/Power Electronics/IGBT  Ron=1e-3  Lon=0  Vf=1  Tf=0  Tt=0  IC=0  Rs=200  Cs=0.1e-6  Measurements=off
  IGBT1 : powerlib/Power Electronics/IGBT  Ron=1e-3  Lon=0  Vf=1  Tf=0  Tt=0  IC=0  Rs=200  Cs=0.1e-6  Measurements=off
  V+ : PMIOPort  Tag=PMCPort  Port=1  Side=Left
  V- : PMIOPort  Tag=PMCPort  Port=2  Side=Left
  C1 : PMIOPort  Tag=PMCPort  Port=3  Side=Right
  C2 : PMIOPort  Tag=PMCPort  Port=4  Side=Right
  wires:
  G/1 -> IGBT/1, IGBT1/1
  connections:
  IGBT1/RConn1 -- D1/LConn1 -- V-/RConn1
  C2/RConn1 -- IGBT1/LConn1 -- D/LConn1
  C1/RConn1 -- D1/RConn1 -- IGBT/RConn1
  D/RConn1 -- V+/RConn1 -- IGBT/LConn1

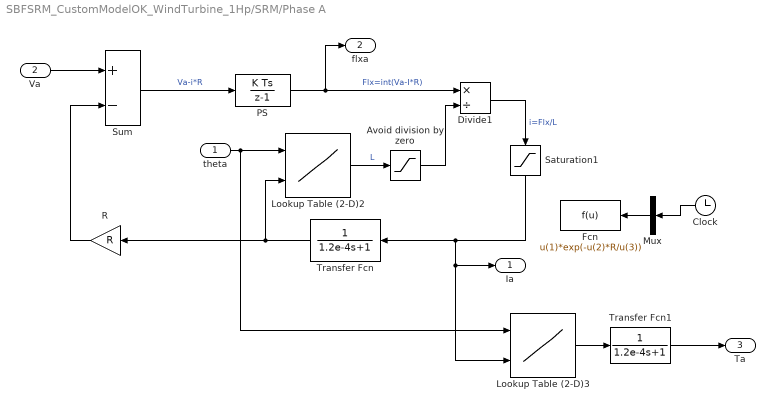
== system SBFSRM_CustomModelOK_WindTurbine_1Hp/SRM/Phase A ==
  theta : Inport
  Va : Inport  Port=2
  "Avoid division by zero " : Saturate  UpperLimit=0.008  LowerLimit=0.001
  Clock : Clock
  Divide1 : Product  Inputs=*/
  Fcn : Fcn  Expr=u(1)*exp(-u(2)*R/u(3))
  Lookup Table (2-D)2 : Lookup2D  RowIndex=[0,1,2,3,4,5,6,7,8,9,10,11,12,13,14,15,16,17,18,19,20,21,22,23,24,25,26,27,28,29,30,31,32,33,34,35,36,37,38,39,40,41,42,43,44,45,46,47,48,49,50,51,52,53,54,55,56,57,58,59,60,61,62,63,64,65,66,67,68,69,70,71,72,73,74,75,76,77,78,79,80,81,82,83,84,85,86,87,88,89,90]  ColumnIndex=[0,0.1,0.3,0.5,0.7,0.9,1,2,3,4,5,6,7,8,9,10,11,12,13,14,15,16,17,18,19,20,21,22,23,24,25,26,27,28,29,30,31,32,33,34,35,36,37,38,39,40,41,42,43,44,45,46,47,48,49,50,51,52,53,54,55,56,57,58,59,60,61,62,63,64,65,66,67,68,69,70,71,72,73,74,75,76,77,78,79,80,81,82,83,84,85,86,87,88,89,90,91,92,93,94,95,96,97,98,99,100,101,102,103,104,105,106,107,108,109,110,111,112,113,114,115,116,117,118,119,120,121,122,123,124,125,126,127,128,129,130,131,132,133,134,135,136,137,138,139,140,141,142,143,144,145,146,147,148,149,150,151,152,153,154,155,156,157,158,159,160,161,162,163,164,165,166,167,168]  Table=InductanceTest
  Lookup Table (2-D)3 : Lookup2D  RowIndex=[0:1:90]  ColumnIndex=[0,1,2,3,4,5,6,7,8,9,10,11,12,13,14,15,16,17,18,19,20,21,22,23,24,25,26,27,28,29,30,31,32,33,34,35,36,37,38,39,40,41,42,43,44,45,46,47,48,49,50,51,52,53,54,55,56,57,58,59,60,61,62,63,64,65,66,67,68,69,70,71,72,73,74,75,76,77,78,79,80,81,82,83,84,85,86,87,88,89,90,91,92,93,94,95,96,97,98,99,100,101,102,103,104,105,106,107,108,109,110,111,112,113,114,115,116,117,118,119,120,121,122,123,124,125,126,127,128,129,130,131,132,133,134,135,136,137,138,139,140,141,142,143,144,145,146,147,148,149,150,151,152,153,154,155,156,157,158,159,160,161,162,163,164,165,166,167,168]  Table=TorqueTest
  Mux : Mux  Inputs=3
  PS : DiscreteIntegrator  SampleTime=Ts  LimitOutput=on  LowerSaturationLimit=0  ICPrevOutput=DiscIntNeverNeededParam  ICPrevScaledInput=DiscIntNeverNeededParam
  R : Gain  Gain=R
  Saturation1 : Saturate  UpperLimit=250  LowerLimit=0
  Sum : Sum  Inputs=+-
  Transfer Fcn : TransferFcn  Denominator=[1.2e-4 1]
  Transfer Fcn1 : TransferFcn  Denominator=[1.2e-4 1]
  Ia : Outport
  flxa : Outport  Port=2
  Ta : Outport  Port=3
  wires:
  Va/1 -> Sum/1
  R/1 -> Sum/2
  Sum/1 -> PS/1  "Va-i*R"
  PS/1 -> Divide1/1, flxa/1  "Flx=int(Va-I*R)"
  theta/1 -> Lookup Table (2-D)2/1, Lookup Table (2-D)3/1
  Lookup Table (2-D)3/1 -> Transfer Fcn1/1
  Divide1/1 -> Saturation1/1  "i=Flx/L"
  Transfer Fcn1/1 -> Ta/1
  Lookup Table (2-D)2/1 -> "Avoid division by zero "/1  "L"
  "Avoid division by zero "/1 -> Divide1/2
  Clock/1 -> Mux/2
  Mux/1 -> Fcn/1
  Saturation1/1 -> Transfer Fcn/1, Ia/1, Lookup Table (2-D)3/2
  Transfer Fcn/1 -> R/1, Lookup Table (2-D)2/2

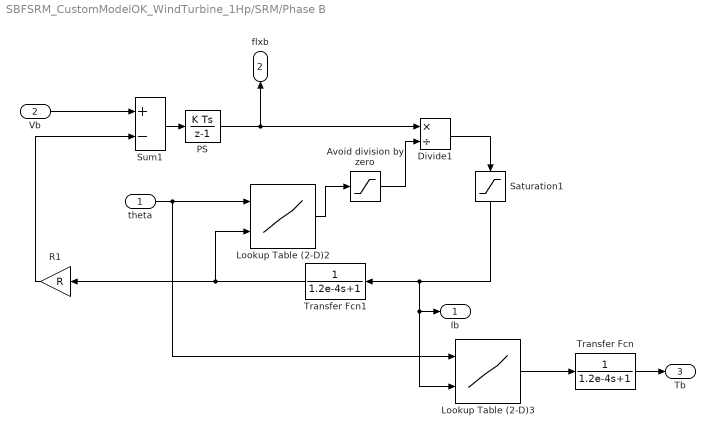
== system SBFSRM_CustomModelOK_WindTurbine_1Hp/SRM/Phase B ==
  theta : Inport
  Vb : Inport  Port=2
  "Avoid division by zero " : Saturate  UpperLimit=0.008  LowerLimit=0.001
  Divide1 : Product  Inputs=*/
  Lookup Table (2-D)2 : Lookup2D  RowIndex=[0,1,2,3,4,5,6,7,8,9,10,11,12,13,14,15,16,17,18,19,20,21,22,23,24,25,26,27,28,29,30,31,32,33,34,35,36,37,38,39,40,41,42,43,44,45,46,47,48,49,50,51,52,53,54,55,56,57,58,59,60,61,62,63,64,65,66,67,68,69,70,71,72,73,74,75,76,77,78,79,80,81,82,83,84,85,86,87,88,89,90]  ColumnIndex=[0,0.1,0.3,0.5,0.7,0.9,1,2,3,4,5,6,7,8,9,10,11,12,13,14,15,16,17,18,19,20,21,22,23,24,25,26,27,28,29,30,31,32,33,34,35,36,37,38,39,40,41,42,43,44,45,46,47,48,49,50,51,52,53,54,55,56,57,58,59,60,61,62,63,64,65,66,67,68,69,70,71,72,73,74,75,76,77,78,79,80,81,82,83,84,85,86,87,88,89,90,91,92,93,94,95,96,97,98,99,100,101,102,103,104,105,106,107,108,109,110,111,112,113,114,115,116,117,118,119,120,121,122,123,124,125,126,127,128,129,130,131,132,133,134,135,136,137,138,139,140,141,142,143,144,145,146,147,148,149,150,151,152,153,154,155,156,157,158,159,160,161,162,163,164,165,166,167,168]  Table=InductanceTest
  Lookup Table (2-D)3 : Lookup2D  RowIndex=[0:1:90]  ColumnIndex=[0,1,2,3,4,5,6,7,8,9,10,11,12,13,14,15,16,17,18,19,20,21,22,23,24,25,26,27,28,29,30,31,32,33,34,35,36,37,38,39,40,41,42,43,44,45,46,47,48,49,50,51,52,53,54,55,56,57,58,59,60,61,62,63,64,65,66,67,68,69,70,71,72,73,74,75,76,77,78,79,80,81,82,83,84,85,86,87,88,89,90,91,92,93,94,95,96,97,98,99,100,101,102,103,104,105,106,107,108,109,110,111,112,113,114,115,116,117,118,119,120,121,122,123,124,125,126,127,128,129,130,131,132,133,134,135,136,137,138,139,140,141,142,143,144,145,146,147,148,149,150,151,152,153,154,155,156,157,158,159,160,161,162,163,164,165,166,167,168]  Table=TorqueTest
  PS : DiscreteIntegrator  SampleTime=Ts  LimitOutput=on  LowerSaturationLimit=0  ICPrevOutput=DiscIntNeverNeededParam  ICPrevScaledInput=DiscIntNeverNeededParam
  R1 : Gain  Gain=R
  Saturation1 : Saturate  UpperLimit=250  LowerLimit=0
  Sum1 : Sum  Inputs=+-
  Transfer Fcn : TransferFcn  Denominator=[1.2e-4 1]
  Transfer Fcn1 : TransferFcn  Denominator=[1.2e-4 1]
  Ib : Outport
  flxb : Outport  Port=2
  Tb : Outport  Port=3
  wires:
  R1/1 -> Sum1/2
  Sum1/1 -> PS/1
  PS/1 -> Divide1/1, flxb/1
  Lookup Table (2-D)3/1 -> Transfer Fcn/1
  Divide1/1 -> Saturation1/1
  Transfer Fcn1/1 -> R1/1, Lookup Table (2-D)2/2
  Saturation1/1 -> Lookup Table (2-D)3/2, Ib/1, Transfer Fcn1/1
  Transfer Fcn/1 -> Tb/1
  Lookup Table (2-D)2/1 -> "Avoid division by zero "/1
  "Avoid division by zero "/1 -> Divide1/2
  theta/1 -> Lookup Table (2-D)3/1, Lookup Table (2-D)2/1
  Vb/1 -> Sum1/1

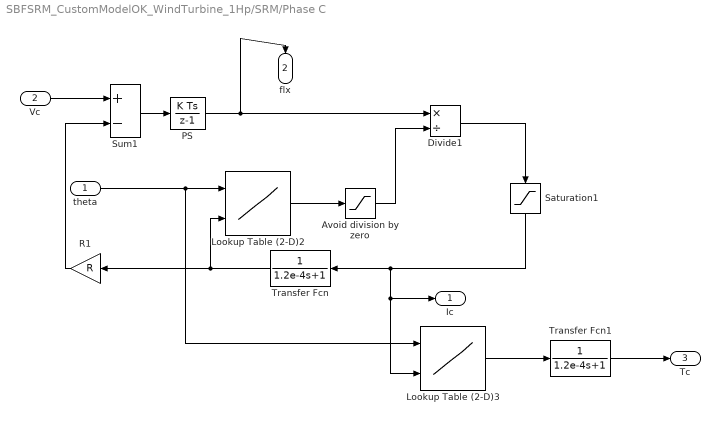
== system SBFSRM_CustomModelOK_WindTurbine_1Hp/SRM/Phase C ==
  theta : Inport
  Vc : Inport  Port=2
  "Avoid division by zero " : Saturate  UpperLimit=0.008  LowerLimit=0.001
  Divide1 : Product  Inputs=*/
  Lookup Table (2-D)2 : Lookup2D  RowIndex=[0,1,2,3,4,5,6,7,8,9,10,11,12,13,14,15,16,17,18,19,20,21,22,23,24,25,26,27,28,29,30,31,32,33,34,35,36,37,38,39,40,41,42,43,44,45,46,47,48,49,50,51,52,53,54,55,56,57,58,59,60,61,62,63,64,65,66,67,68,69,70,71,72,73,74,75,76,77,78,79,80,81,82,83,84,85,86,87,88,89,90]  ColumnIndex=[0,0.1,0.3,0.5,0.7,0.9,1,2,3,4,5,6,7,8,9,10,11,12,13,14,15,16,17,18,19,20,21,22,23,24,25,26,27,28,29,30,31,32,33,34,35,36,37,38,39,40,41,42,43,44,45,46,47,48,49,50,51,52,53,54,55,56,57,58,59,60,61,62,63,64,65,66,67,68,69,70,71,72,73,74,75,76,77,78,79,80,81,82,83,84,85,86,87,88,89,90,91,92,93,94,95,96,97,98,99,100,101,102,103,104,105,106,107,108,109,110,111,112,113,114,115,116,117,118,119,120,121,122,123,124,125,126,127,128,129,130,131,132,133,134,135,136,137,138,139,140,141,142,143,144,145,146,147,148,149,150,151,152,153,154,155,156,157,158,159,160,161,162,163,164,165,166,167,168]  Table=InductanceTest
  Lookup Table (2-D)3 : Lookup2D  RowIndex=[0:1:90]  ColumnIndex=[0,1,2,3,4,5,6,7,8,9,10,11,12,13,14,15,16,17,18,19,20,21,22,23,24,25,26,27,28,29,30,31,32,33,34,35,36,37,38,39,40,41,42,43,44,45,46,47,48,49,50,51,52,53,54,55,56,57,58,59,60,61,62,63,64,65,66,67,68,69,70,71,72,73,74,75,76,77,78,79,80,81,82,83,84,85,86,87,88,89,90,91,92,93,94,95,96,97,98,99,100,101,102,103,104,105,106,107,108,109,110,111,112,113,114,115,116,117,118,119,120,121,122,123,124,125,126,127,128,129,130,131,132,133,134,135,136,137,138,139,140,141,142,143,144,145,146,147,148,149,150,151,152,153,154,155,156,157,158,159,160,161,162,163,164,165,166,167,168]  Table=TorqueTest
  PS : DiscreteIntegrator  SampleTime=Ts  LimitOutput=on  LowerSaturationLimit=0  ICPrevOutput=DiscIntNeverNeededParam  ICPrevScaledInput=DiscIntNeverNeededParam
  R1 : Gain  Gain=R
  Saturation1 : Saturate  UpperLimit=250  LowerLimit=0
  Sum1 : Sum  Inputs=+-
  Transfer Fcn : TransferFcn  Denominator=[1.2e-4 1]
  Transfer Fcn1 : TransferFcn  Denominator=[1.2e-4 1]
  Ic : Outport
  flx : Outport  Port=2
  Tc : Outport  Port=3
  wires:
  R1/1 -> Sum1/2
  Sum1/1 -> PS/1
  PS/1 -> flx/1, Divide1/1
  Vc/1 -> Sum1/1
  theta/1 -> Lookup Table (2-D)3/1, Lookup Table (2-D)2/1
  Lookup Table (2-D)3/1 -> Transfer Fcn1/1
  Divide1/1 -> Saturation1/1
  Saturation1/1 -> Ic/1, Lookup Table (2-D)3/2, Transfer Fcn/1
  Transfer Fcn/1 -> R1/1, Lookup Table (2-D)2/2
  Transfer Fcn1/1 -> Tc/1
  Lookup Table (2-D)2/1 -> "Avoid division by zero "/1
  "Avoid division by zero "/1 -> Divide1/2

== matlab function Dwell Angle Generation/MATLAB Function ==
  data: ang input double; y1 output double; y2 output double
function [y1,y2] = fcn(ang)
%#codegen
alfa=ang(1);
beta=ang(2);
y1=0;
if alfa>beta
    y1=0;
    y2=alfa;
else
    y1=alfa;
    y2=60;   
end
end
